simulink model "truck_state_space_model"  (R2013b)
settings: Solver=ode15s  StartTime=0.0  StopTime=10.0  RelTol=1e-16
values from neighbouring files (symbols this model uses):
  A = aak1+aak2+aak3+aak4+aak5+aak6    [truck_force.m]
  C = fk/max(A)    [truck_force.m]
  dyk = 0.007    [truck.m]    (also in truck_sis.m)
  Vk = 25    [truck.m]    (also in truck_sis.m = 16.6666666667)
  wk = Vk/dyk    (= 3571.42857143)    [truck.m]    (also in truck_sis.m = 2380.95238095)
undefined symbols (not defined in the file or in its folder): B, D, l_1, l_2, l_3
settings Model: Creator=user  LastModifiedBy=user

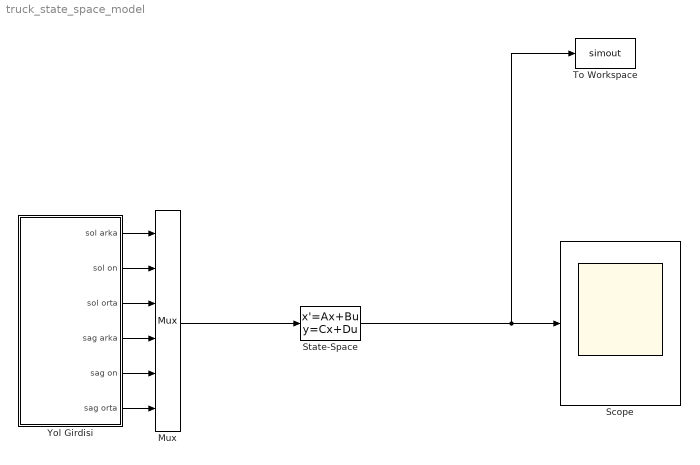
== system truck_state_space_model ==
  Mux : Mux  Inputs=6
  Scope : Scope
      settings: ShowLegends=on  YMin=-0.07  YMax=0.07  MaxDataPoints=500000
  State-Space : StateSpace  A=A  B=B  C=C  D=D  X0=0
  To Workspace : ToWorkspace  VariableName=simout  SampleTime=-1  SaveFormat=Timeseries
  Yol Girdisi : Subsystem
  wires:
  State-Space/1 -> To Workspace/1, Scope/1
  Mux/1 -> State-Space/1
  Yol Girdisi/1(sol arka) -> Mux/1
  Yol Girdisi/2(sol on) -> Mux/2
  Yol Girdisi/3(sol orta) -> Mux/3
  Yol Girdisi/4(sag arka) -> Mux/4
  Yol Girdisi/5(sag on) -> Mux/5
  Yol Girdisi/6(sag orta) -> Mux/6

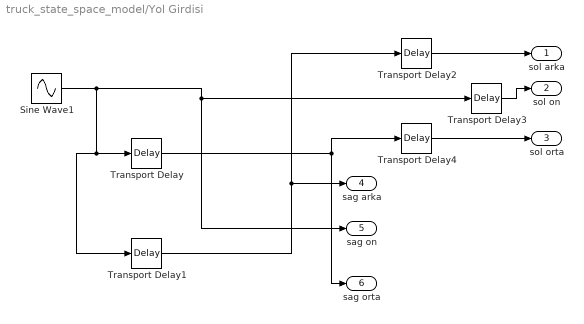
== system truck_state_space_model/Yol Girdisi ==
  Sine Wave1 : Sin  Amplitude=dyk  Frequency=wk  SampleTime=0
  Transport Delay : TransportDelay  DelayTime=(l_2+l_3)/Vk
  Transport Delay1 : TransportDelay  DelayTime=(l_1+l_2)/Vk
  Transport Delay2 : TransportDelay  DelayTime=0.001
  Transport Delay3 : TransportDelay  DelayTime=0.001
  Transport Delay4 : TransportDelay  DelayTime=0.001
  sol arka : Outport
  sol on : Outport  Port=2
  sol orta : Outport  Port=3
  sag arka : Outport  Port=4
  sag on : Outport  Port=5
  sag orta : Outport  Port=6
  wires:
  Sine Wave1/1 -> sag on/1, Transport Delay3/1, Transport Delay/1, Transport Delay1/1
  Transport Delay/1 -> sag orta/1, Transport Delay4/1
  Transport Delay1/1 -> sag arka/1, Transport Delay2/1
  Transport Delay2/1 -> sol arka/1
  Transport Delay3/1 -> sol on/1
  Transport Delay4/1 -> sol orta/1
